simulink model "task1"  (Simulink 10.3)
settings: Solver=ode45  StartTime=0.0  StopTime=10.0  RelTol=1e-3  EnableMultiTasking=on
settings Model: Creator=ADMIN  LastModifiedBy=Safi Ullah
settings DataIOCC: LimitDataPoints=on
settings DebuggingCC: SolverPrmCheckMsg=warning

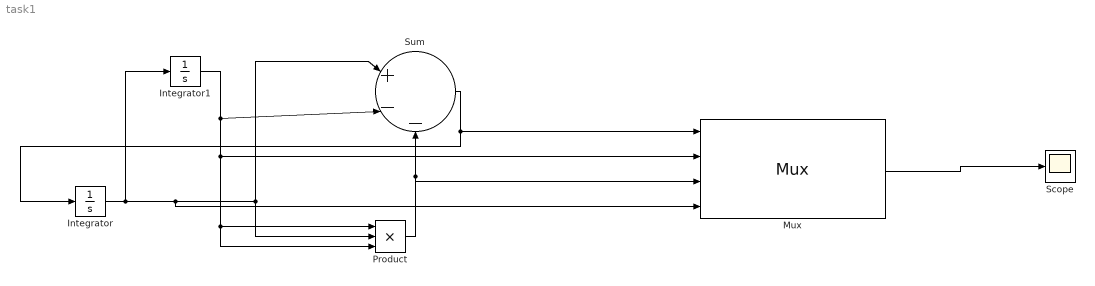
== system task1 ==
  Integrator : Integrator  InitialCondition=[0 1]
  Integrator1 : Integrator  InitialCondition=[0 1]
  Mux : Mux
  Product : Product  Inputs=3  RndMeth=Zero
  Scope : Scope
  Sum : Sum  Inputs=|+--
  wires:
  Integrator/1 -> Integrator1/1, Sum/1, Product/2, Mux/4
  Integrator1/1 -> Sum/2, Product/1, Product/3, Mux/2
  Product/1 -> Sum/3, Mux/3
  Sum/1 -> Integrator/1, Mux/1
  Mux/1 -> Scope/1
